simulink model "TST_ASDrf_Governor"  (R2016b)
settings: Solver=FixedStepDiscrete  StartTime=0.0  StopTime=simTime  FixedStep=sampleTime  RelTol=1e-3
values from neighbouring files (symbols this model uses):
  testCase = 1    [initTST_ASDrf_Governor_001.m]    (also in initTST_ASDrf_Governor_002.m = 2; initTST_ASDrf_Governor_003.m = 3)
libraries: simulink x10, UnitTest_Lib x6
settings Model: Creator=zhengjinyan  LastModifiedBy=zhengjinyan
settings DebuggingCC: SignalRangeChecking=error

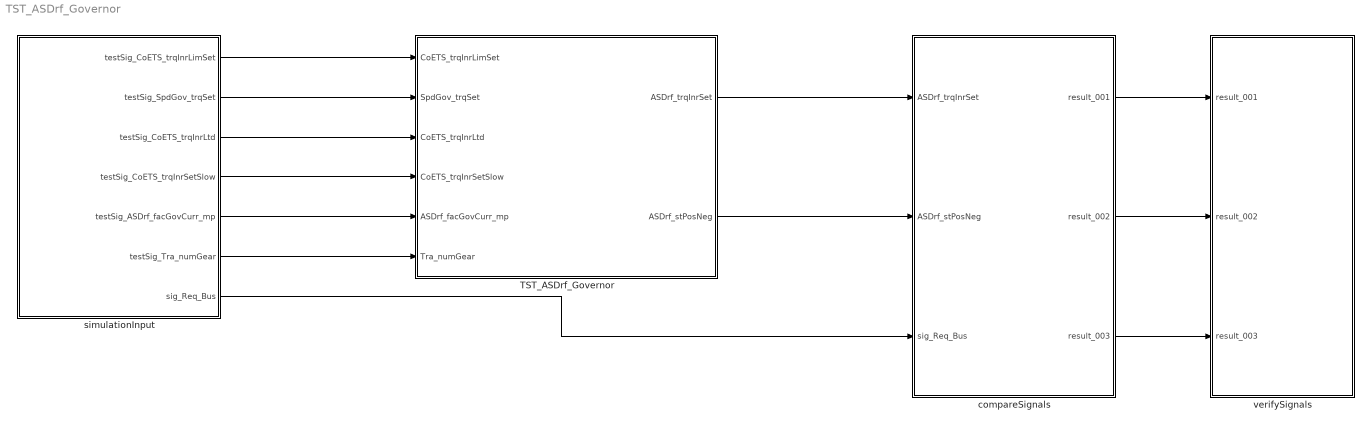
== system TST_ASDrf_Governor ==
  TST_ASDrf_Governor : Subsystem
  compareSignals : Subsystem
  simulationInput : Subsystem
  verifySignals : Subsystem
  wires:
  simulationInput/1(testSig_CoETS_trqInrLimSet) -> TST_ASDrf_Governor/1(CoETS_trqInrLimSet)
  simulationInput/2(testSig_SpdGov_trqSet) -> TST_ASDrf_Governor/2(SpdGov_trqSet)
  simulationInput/3(testSig_CoETS_trqInrLtd) -> TST_ASDrf_Governor/3(CoETS_trqInrLtd)
  simulationInput/4(testSig_CoETS_trqInrSetSlow) -> TST_ASDrf_Governor/4(CoETS_trqInrSetSlow)
  simulationInput/5(testSig_ASDrf_facGovCurr_mp) -> TST_ASDrf_Governor/5(ASDrf_facGovCurr_mp)
  simulationInput/6(testSig_Tra_numGear) -> TST_ASDrf_Governor/6(Tra_numGear)
  TST_ASDrf_Governor/1(ASDrf_trqInrSet) -> compareSignals/1(ASDrf_trqInrSet)
  TST_ASDrf_Governor/2(ASDrf_stPosNeg) -> compareSignals/2(ASDrf_stPosNeg)
  simulationInput/7(sig_Req_Bus) -> compareSignals/3(sig_Req_Bus)
  compareSignals/1(result_001) -> verifySignals/1(result_001)
  compareSignals/2(result_002) -> verifySignals/2(result_002)
  compareSignals/3(result_003) -> verifySignals/3(result_003)

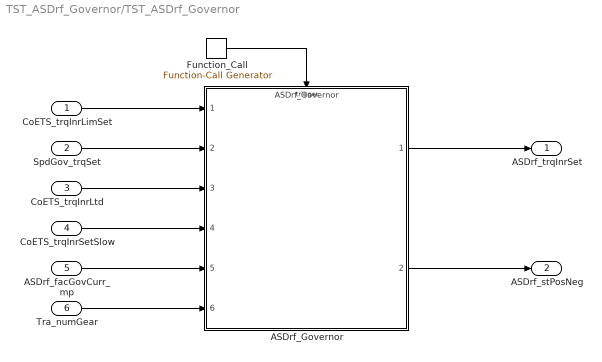
== system TST_ASDrf_Governor/TST_ASDrf_Governor ==
  CoETS_trqInrLimSet : Inport
  SpdGov_trqSet : Inport  Port=2
  CoETS_trqInrLtd : Inport  Port=3
  CoETS_trqInrSetSlow : Inport  Port=4
  ASDrf_facGovCurr_mp : Inport  Port=5
  Tra_numGear : Inport  Port=6
  ASDrf_Governor : ModelReference  ModelNameDialog=ASDrf_Governor  SimulationMode=Normal  ModelReferenceVersion=1.11  TriggerPortName=function  TriggerPortTriggerType=function-call  TriggerPortStatesWhenEnabling=held
  Function_Call : simulink/Ports & Subsystems/Function-Call Generator  sample_time=sampleTime  numberOfIterations=1
  ASDrf_trqInrSet : Outport
  ASDrf_stPosNeg : Outport  Port=2
  wires:
  Function_Call/1 -> ASDrf_Governor/Trigger
  CoETS_trqInrLimSet/1 -> ASDrf_Governor/1
  SpdGov_trqSet/1 -> ASDrf_Governor/2
  CoETS_trqInrLtd/1 -> ASDrf_Governor/3
  CoETS_trqInrSetSlow/1 -> ASDrf_Governor/4
  ASDrf_facGovCurr_mp/1 -> ASDrf_Governor/5
  Tra_numGear/1 -> ASDrf_Governor/6
  ASDrf_Governor/1 -> ASDrf_trqInrSet/1
  ASDrf_Governor/2 -> ASDrf_stPosNeg/1

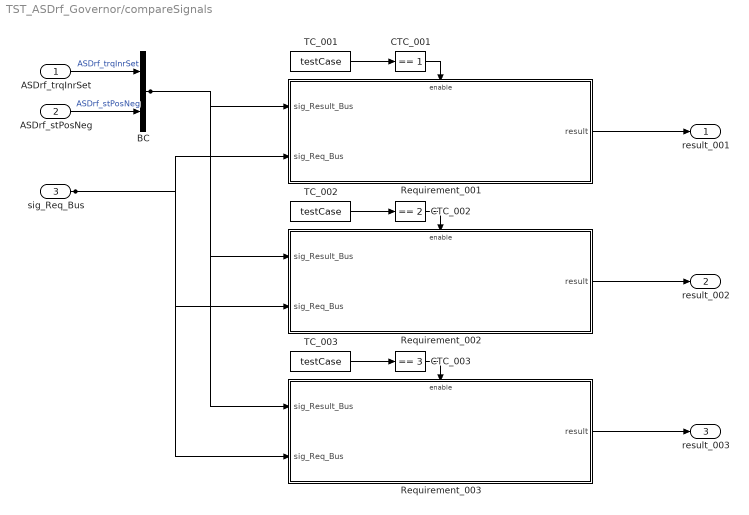
== system TST_ASDrf_Governor/compareSignals ==
  ASDrf_trqInrSet : Inport
  ASDrf_stPosNeg : Inport  Port=2
  sig_Req_Bus : Inport  Port=3
  BC : BusCreator  Inputs=2
  CTC_001 : simulink/Logic and Bit Operations/Compare To Constant  relop===  const=1  OutDataTypeStr=boolean
  CTC_002 : simulink/Logic and Bit Operations/Compare To Constant  relop===  const=2  OutDataTypeStr=boolean
  CTC_003 : simulink/Logic and Bit Operations/Compare To Constant  relop===  const=3  OutDataTypeStr=boolean
  Requirement_001 : Subsystem
  Requirement_002 : Subsystem
  Requirement_003 : Subsystem
  TC_001 : Constant  Value=testCase
  TC_002 : Constant  Value=testCase
  TC_003 : Constant  Value=testCase
  result_001 : Outport
  result_002 : Outport  Port=2
  result_003 : Outport  Port=3
  wires:
  ASDrf_trqInrSet/1 -> BC/1  "ASDrf_trqInrSet"
  ASDrf_stPosNeg/1 -> BC/2  "ASDrf_stPosNeg"
  TC_001/1 -> CTC_001/1
  CTC_001/1 -> Requirement_001/Enable
  sig_Req_Bus/1 -> Requirement_001/2(sig_Req_Bus), Requirement_002/2(sig_Req_Bus), Requirement_003/2(sig_Req_Bus)
  BC/1 -> Requirement_001/1(sig_Result_Bus), Requirement_002/1(sig_Result_Bus), Requirement_003/1(sig_Result_Bus)
  Requirement_001/1(result) -> result_001/1
  TC_002/1 -> CTC_002/1
  CTC_002/1 -> Requirement_002/Enable
  Requirement_002/1(result) -> result_002/1
  TC_003/1 -> CTC_003/1
  CTC_003/1 -> Requirement_003/Enable
  Requirement_003/1(result) -> result_003/1

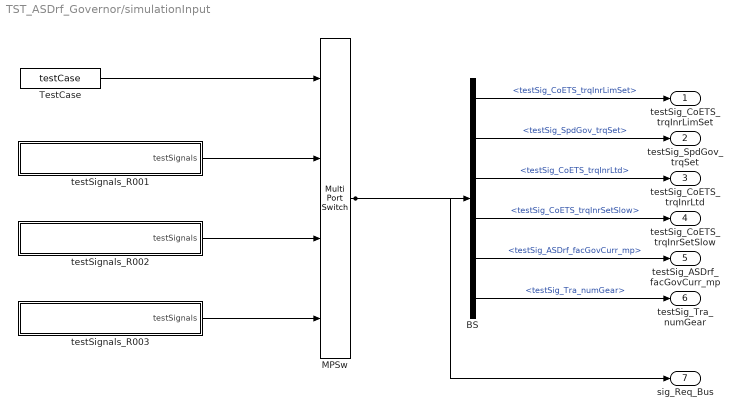
== system TST_ASDrf_Governor/simulationInput ==
  BS : BusSelector  OutputSignals=testSig_CoETS_trqInrLimSet,testSig_SpdGov_trqSet,testSig_CoETS_trqInrLtd,testSig_CoETS_trqInrSetSlow,testSig_ASDrf_facGovCurr_mp,testSig_Tra_numGear
  MPSw : MultiPortSwitch  SaturateOnIntegerOverflow=on  InputSameDT=on
  TestCase : Constant  Value=testCase
  testSignals_R001 : Subsystem
  testSignals_R002 : Subsystem
  testSignals_R003 : Subsystem
  testSig_CoETS_trqInrLimSet : Outport
  testSig_SpdGov_trqSet : Outport  Port=2
  testSig_CoETS_trqInrLtd : Outport  Port=3
  testSig_CoETS_trqInrSetSlow : Outport  Port=4
  testSig_ASDrf_facGovCurr_mp : Outport  Port=5
  testSig_Tra_numGear : Outport  Port=6
  sig_Req_Bus : Outport  Port=7
  wires:
  BS/1 -> testSig_CoETS_trqInrLimSet/1  "<testSig_CoETS_trqInrLimSet>"
  BS/2 -> testSig_SpdGov_trqSet/1  "<testSig_SpdGov_trqSet>"
  BS/3 -> testSig_CoETS_trqInrLtd/1  "<testSig_CoETS_trqInrLtd>"
  BS/4 -> testSig_CoETS_trqInrSetSlow/1  "<testSig_CoETS_trqInrSetSlow>"
  BS/5 -> testSig_ASDrf_facGovCurr_mp/1  "<testSig_ASDrf_facGovCurr_mp>"
  BS/6 -> testSig_Tra_numGear/1  "<testSig_Tra_numGear>"
  MPSw/1 -> BS/1, sig_Req_Bus/1
  TestCase/1 -> MPSw/1
  testSignals_R001/1(testSignals) -> MPSw/2
  testSignals_R002/1(testSignals) -> MPSw/3
  testSignals_R003/1(testSignals) -> MPSw/4

== system TST_ASDrf_Governor/verifySignals ==
  result_001 : Inport
  result_002 : Inport  Port=2
  result_003 : Inport  Port=3
  Assertion_001 : Assertion  Enabled=off
  Assertion_002 : Assertion  Enabled=off
  Assertion_003 : Assertion  Enabled=off
  wires:
  result_001/1 -> Assertion_001/1
  result_002/1 -> Assertion_002/1
  result_003/1 -> Assertion_003/1

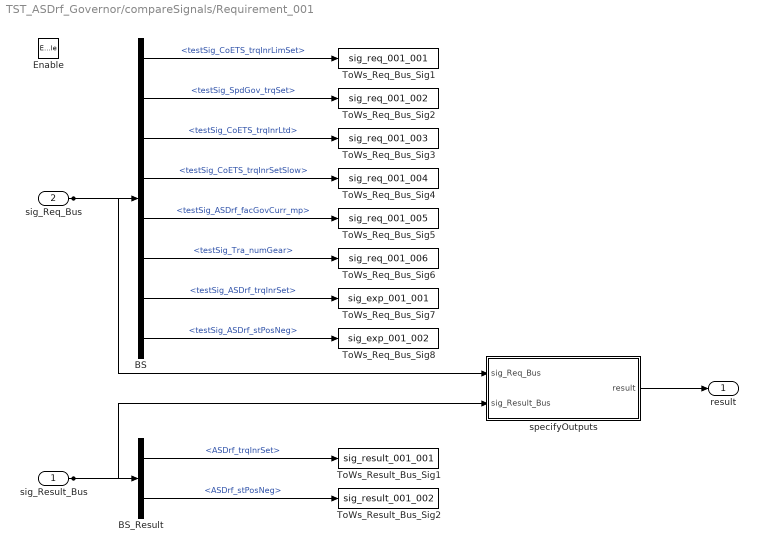
== system TST_ASDrf_Governor/compareSignals/Requirement_001 ==
  sig_Result_Bus : Inport
  sig_Req_Bus : Inport  Port=2
  Enable : EnablePort
  BS : BusSelector  OutputSignals=testSig_CoETS_trqInrLimSet,testSig_SpdGov_trqSet,testSig_CoETS_trqInrLtd,testSig_CoETS_trqInrSetSlow,testSig_ASDrf_facGovCurr_mp,testSig_Tra_numGear,testSig_ASDrf_trqInrSet,testSig_ASDrf_stPosNeg
  BS_Result : BusSelector  OutputSignals=ASDrf_trqInrSet,ASDrf_stPosNeg
  ToWs_Req_Bus_Sig1 : ToWorkspace  VariableName=sig_req_001_001  SaveFormat=Structure With Time
  ToWs_Req_Bus_Sig2 : ToWorkspace  VariableName=sig_req_001_002  SaveFormat=Structure With Time
  ToWs_Req_Bus_Sig3 : ToWorkspace  VariableName=sig_req_001_003  SaveFormat=Structure With Time
  ToWs_Req_Bus_Sig4 : ToWorkspace  VariableName=sig_req_001_004  SaveFormat=Structure With Time
  ToWs_Req_Bus_Sig5 : ToWorkspace  VariableName=sig_req_001_005  SaveFormat=Structure With Time
  ToWs_Req_Bus_Sig6 : ToWorkspace  VariableName=sig_req_001_006  SaveFormat=Structure With Time
  ToWs_Req_Bus_Sig7 : ToWorkspace  VariableName=sig_exp_001_001  SaveFormat=Structure With Time
  ToWs_Req_Bus_Sig8 : ToWorkspace  VariableName=sig_exp_001_002  SaveFormat=Structure With Time
  ToWs_Result_Bus_Sig1 : ToWorkspace  VariableName=sig_result_001_001  SaveFormat=Structure With Time
  ToWs_Result_Bus_Sig2 : ToWorkspace  VariableName=sig_result_001_002  SaveFormat=Structure With Time
  specifyOutputs : Subsystem
  result : Outport
  wires:
  sig_Req_Bus/1 -> BS/1, specifyOutputs/1(sig_Req_Bus)
  BS/1 -> ToWs_Req_Bus_Sig1/1  "<testSig_CoETS_trqInrLimSet>"
  BS/2 -> ToWs_Req_Bus_Sig2/1  "<testSig_SpdGov_trqSet>"
  BS/3 -> ToWs_Req_Bus_Sig3/1  "<testSig_CoETS_trqInrLtd>"
  BS/4 -> ToWs_Req_Bus_Sig4/1  "<testSig_CoETS_trqInrSetSlow>"
  BS/5 -> ToWs_Req_Bus_Sig5/1  "<testSig_ASDrf_facGovCurr_mp>"
  BS/6 -> ToWs_Req_Bus_Sig6/1  "<testSig_Tra_numGear>"
  BS/7 -> ToWs_Req_Bus_Sig7/1  "<testSig_ASDrf_trqInrSet>"
  BS/8 -> ToWs_Req_Bus_Sig8/1  "<testSig_ASDrf_stPosNeg>"
  sig_Result_Bus/1 -> BS_Result/1, specifyOutputs/2(sig_Result_Bus)
  BS_Result/1 -> ToWs_Result_Bus_Sig1/1  "<ASDrf_trqInrSet>"
  BS_Result/2 -> ToWs_Result_Bus_Sig2/1  "<ASDrf_stPosNeg>"
  specifyOutputs/1(result) -> result/1

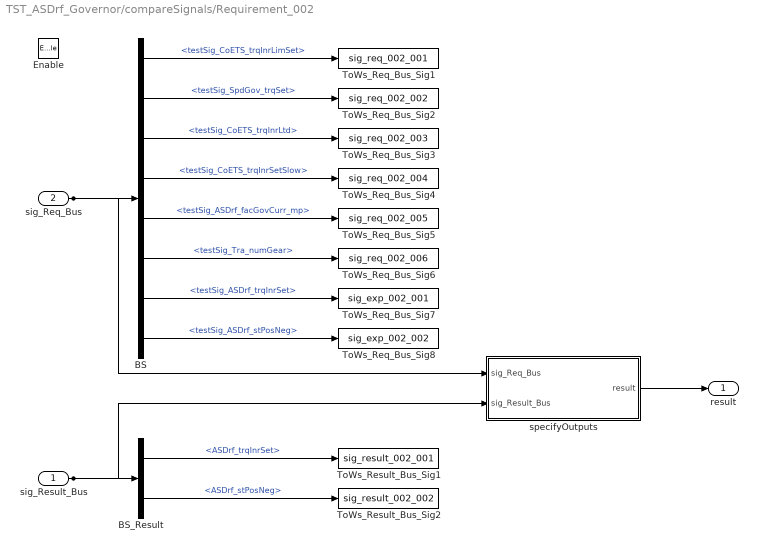
== system TST_ASDrf_Governor/compareSignals/Requirement_002 ==
  sig_Result_Bus : Inport
  sig_Req_Bus : Inport  Port=2
  Enable : EnablePort
  BS : BusSelector  OutputSignals=testSig_CoETS_trqInrLimSet,testSig_SpdGov_trqSet,testSig_CoETS_trqInrLtd,testSig_CoETS_trqInrSetSlow,testSig_ASDrf_facGovCurr_mp,testSig_Tra_numGear,testSig_ASDrf_trqInrSet,testSig_ASDrf_stPosNeg
  BS_Result : BusSelector  OutputSignals=ASDrf_trqInrSet,ASDrf_stPosNeg
  ToWs_Req_Bus_Sig1 : ToWorkspace  VariableName=sig_req_002_001  SaveFormat=Structure With Time
  ToWs_Req_Bus_Sig2 : ToWorkspace  VariableName=sig_req_002_002  SaveFormat=Structure With Time
  ToWs_Req_Bus_Sig3 : ToWorkspace  VariableName=sig_req_002_003  SaveFormat=Structure With Time
  ToWs_Req_Bus_Sig4 : ToWorkspace  VariableName=sig_req_002_004  SaveFormat=Structure With Time
  ToWs_Req_Bus_Sig5 : ToWorkspace  VariableName=sig_req_002_005  SaveFormat=Structure With Time
  ToWs_Req_Bus_Sig6 : ToWorkspace  VariableName=sig_req_002_006  SaveFormat=Structure With Time
  ToWs_Req_Bus_Sig7 : ToWorkspace  VariableName=sig_exp_002_001  SaveFormat=Structure With Time
  ToWs_Req_Bus_Sig8 : ToWorkspace  VariableName=sig_exp_002_002  SaveFormat=Structure With Time
  ToWs_Result_Bus_Sig1 : ToWorkspace  VariableName=sig_result_002_001  SaveFormat=Structure With Time
  ToWs_Result_Bus_Sig2 : ToWorkspace  VariableName=sig_result_002_002  SaveFormat=Structure With Time
  specifyOutputs : Subsystem
  result : Outport
  wires:
  sig_Req_Bus/1 -> BS/1, specifyOutputs/1(sig_Req_Bus)
  BS/1 -> ToWs_Req_Bus_Sig1/1  "<testSig_CoETS_trqInrLimSet>"
  BS/2 -> ToWs_Req_Bus_Sig2/1  "<testSig_SpdGov_trqSet>"
  BS/3 -> ToWs_Req_Bus_Sig3/1  "<testSig_CoETS_trqInrLtd>"
  BS/4 -> ToWs_Req_Bus_Sig4/1  "<testSig_CoETS_trqInrSetSlow>"
  BS/5 -> ToWs_Req_Bus_Sig5/1  "<testSig_ASDrf_facGovCurr_mp>"
  BS/6 -> ToWs_Req_Bus_Sig6/1  "<testSig_Tra_numGear>"
  BS/7 -> ToWs_Req_Bus_Sig7/1  "<testSig_ASDrf_trqInrSet>"
  BS/8 -> ToWs_Req_Bus_Sig8/1  "<testSig_ASDrf_stPosNeg>"
  sig_Result_Bus/1 -> BS_Result/1, specifyOutputs/2(sig_Result_Bus)
  BS_Result/1 -> ToWs_Result_Bus_Sig1/1  "<ASDrf_trqInrSet>"
  BS_Result/2 -> ToWs_Result_Bus_Sig2/1  "<ASDrf_stPosNeg>"
  specifyOutputs/1(result) -> result/1

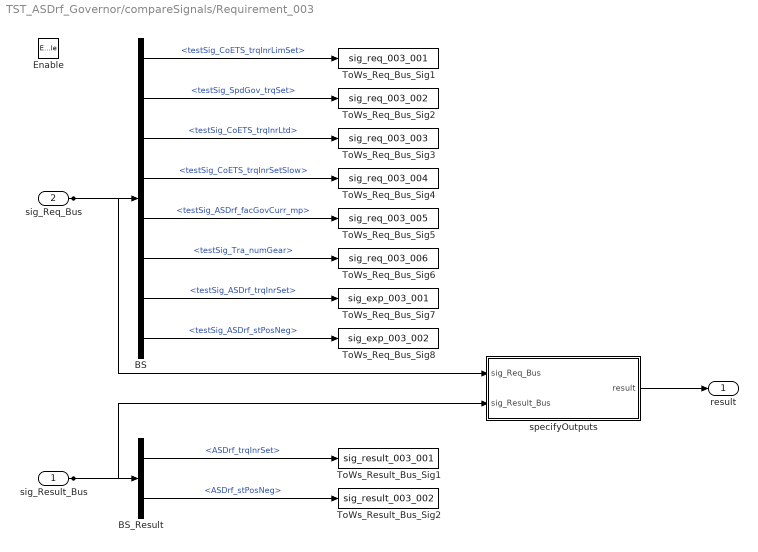
== system TST_ASDrf_Governor/compareSignals/Requirement_003 ==
  sig_Result_Bus : Inport
  sig_Req_Bus : Inport  Port=2
  Enable : EnablePort
  BS : BusSelector  OutputSignals=testSig_CoETS_trqInrLimSet,testSig_SpdGov_trqSet,testSig_CoETS_trqInrLtd,testSig_CoETS_trqInrSetSlow,testSig_ASDrf_facGovCurr_mp,testSig_Tra_numGear,testSig_ASDrf_trqInrSet,testSig_ASDrf_stPosNeg
  BS_Result : BusSelector  OutputSignals=ASDrf_trqInrSet,ASDrf_stPosNeg
  ToWs_Req_Bus_Sig1 : ToWorkspace  VariableName=sig_req_003_001  SaveFormat=Structure With Time
  ToWs_Req_Bus_Sig2 : ToWorkspace  VariableName=sig_req_003_002  SaveFormat=Structure With Time
  ToWs_Req_Bus_Sig3 : ToWorkspace  VariableName=sig_req_003_003  SaveFormat=Structure With Time
  ToWs_Req_Bus_Sig4 : ToWorkspace  VariableName=sig_req_003_004  SaveFormat=Structure With Time
  ToWs_Req_Bus_Sig5 : ToWorkspace  VariableName=sig_req_003_005  SaveFormat=Structure With Time
  ToWs_Req_Bus_Sig6 : ToWorkspace  VariableName=sig_req_003_006  SaveFormat=Structure With Time
  ToWs_Req_Bus_Sig7 : ToWorkspace  VariableName=sig_exp_003_001  SaveFormat=Structure With Time
  ToWs_Req_Bus_Sig8 : ToWorkspace  VariableName=sig_exp_003_002  SaveFormat=Structure With Time
  ToWs_Result_Bus_Sig1 : ToWorkspace  VariableName=sig_result_003_001  SaveFormat=Structure With Time
  ToWs_Result_Bus_Sig2 : ToWorkspace  VariableName=sig_result_003_002  SaveFormat=Structure With Time
  specifyOutputs : Subsystem
  result : Outport
  wires:
  sig_Req_Bus/1 -> BS/1, specifyOutputs/1(sig_Req_Bus)
  BS/1 -> ToWs_Req_Bus_Sig1/1  "<testSig_CoETS_trqInrLimSet>"
  BS/2 -> ToWs_Req_Bus_Sig2/1  "<testSig_SpdGov_trqSet>"
  BS/3 -> ToWs_Req_Bus_Sig3/1  "<testSig_CoETS_trqInrLtd>"
  BS/4 -> ToWs_Req_Bus_Sig4/1  "<testSig_CoETS_trqInrSetSlow>"
  BS/5 -> ToWs_Req_Bus_Sig5/1  "<testSig_ASDrf_facGovCurr_mp>"
  BS/6 -> ToWs_Req_Bus_Sig6/1  "<testSig_Tra_numGear>"
  BS/7 -> ToWs_Req_Bus_Sig7/1  "<testSig_ASDrf_trqInrSet>"
  BS/8 -> ToWs_Req_Bus_Sig8/1  "<testSig_ASDrf_stPosNeg>"
  sig_Result_Bus/1 -> BS_Result/1, specifyOutputs/2(sig_Result_Bus)
  BS_Result/1 -> ToWs_Result_Bus_Sig1/1  "<ASDrf_trqInrSet>"
  BS_Result/2 -> ToWs_Result_Bus_Sig2/1  "<ASDrf_stPosNeg>"
  specifyOutputs/1(result) -> result/1

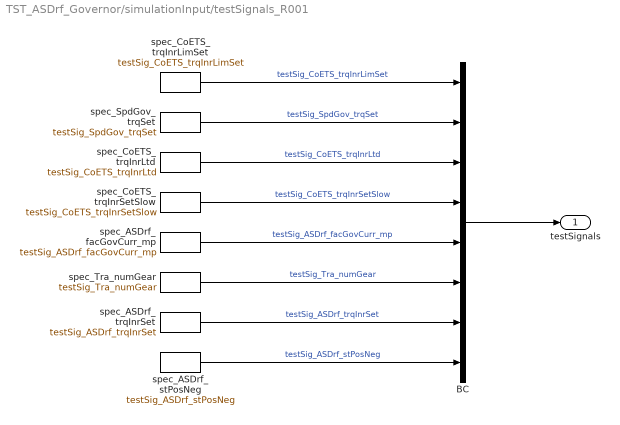
== system TST_ASDrf_Governor/simulationInput/testSignals_R001 ==
  BC : BusCreator  Inputs=8
  spec_ASDrf_facGovCurr_mp : FromWorkspace  VariableName=testSig_ASDrf_facGovCurr_mp  Interpolate=off  OutputAfterFinalValue=Holding final value
  spec_ASDrf_stPosNeg : FromWorkspace  VariableName=testSig_ASDrf_stPosNeg  Interpolate=off  OutputAfterFinalValue=Holding final value
  spec_ASDrf_trqInrSet : FromWorkspace  VariableName=testSig_ASDrf_trqInrSet  Interpolate=off  OutputAfterFinalValue=Holding final value
  spec_CoETS_trqInrLimSet : FromWorkspace  VariableName=testSig_CoETS_trqInrLimSet  Interpolate=off  OutputAfterFinalValue=Holding final value
  spec_CoETS_trqInrLtd : FromWorkspace  VariableName=testSig_CoETS_trqInrLtd  Interpolate=off  OutputAfterFinalValue=Holding final value
  spec_CoETS_trqInrSetSlow : FromWorkspace  VariableName=testSig_CoETS_trqInrSetSlow  Interpolate=off  OutputAfterFinalValue=Holding final value
  spec_SpdGov_trqSet : FromWorkspace  VariableName=testSig_SpdGov_trqSet  Interpolate=off  OutputAfterFinalValue=Holding final value
  spec_Tra_numGear : FromWorkspace  VariableName=testSig_Tra_numGear  Interpolate=off  OutputAfterFinalValue=Holding final value
  testSignals : Outport
  wires:
  BC/1 -> testSignals/1
  spec_CoETS_trqInrLimSet/1 -> BC/1  "testSig_CoETS_trqInrLimSet"
  spec_SpdGov_trqSet/1 -> BC/2  "testSig_SpdGov_trqSet"
  spec_CoETS_trqInrLtd/1 -> BC/3  "testSig_CoETS_trqInrLtd"
  spec_CoETS_trqInrSetSlow/1 -> BC/4  "testSig_CoETS_trqInrSetSlow"
  spec_ASDrf_facGovCurr_mp/1 -> BC/5  "testSig_ASDrf_facGovCurr_mp"
  spec_Tra_numGear/1 -> BC/6  "testSig_Tra_numGear"
  spec_ASDrf_trqInrSet/1 -> BC/7  "testSig_ASDrf_trqInrSet"
  spec_ASDrf_stPosNeg/1 -> BC/8  "testSig_ASDrf_stPosNeg"

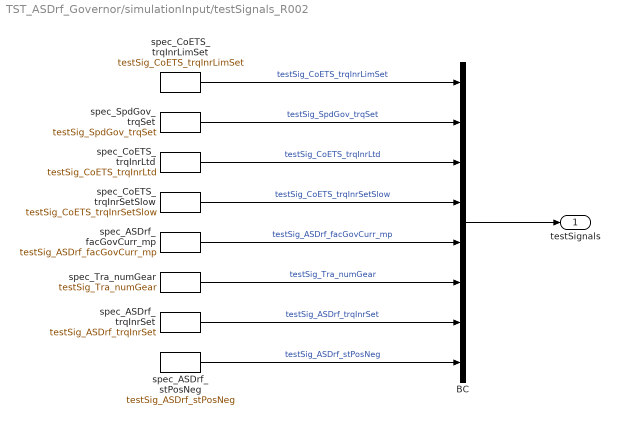
== system TST_ASDrf_Governor/simulationInput/testSignals_R002 ==
  BC : BusCreator  Inputs=8
  spec_ASDrf_facGovCurr_mp : FromWorkspace  VariableName=testSig_ASDrf_facGovCurr_mp  Interpolate=off  OutputAfterFinalValue=Holding final value
  spec_ASDrf_stPosNeg : FromWorkspace  VariableName=testSig_ASDrf_stPosNeg  Interpolate=off  OutputAfterFinalValue=Holding final value
  spec_ASDrf_trqInrSet : FromWorkspace  VariableName=testSig_ASDrf_trqInrSet  Interpolate=off  OutputAfterFinalValue=Holding final value
  spec_CoETS_trqInrLimSet : FromWorkspace  VariableName=testSig_CoETS_trqInrLimSet  Interpolate=off  OutputAfterFinalValue=Holding final value
  spec_CoETS_trqInrLtd : FromWorkspace  VariableName=testSig_CoETS_trqInrLtd  Interpolate=off  OutputAfterFinalValue=Holding final value
  spec_CoETS_trqInrSetSlow : FromWorkspace  VariableName=testSig_CoETS_trqInrSetSlow  Interpolate=off  OutputAfterFinalValue=Holding final value
  spec_SpdGov_trqSet : FromWorkspace  VariableName=testSig_SpdGov_trqSet  Interpolate=off  OutputAfterFinalValue=Holding final value
  spec_Tra_numGear : FromWorkspace  VariableName=testSig_Tra_numGear  Interpolate=off  OutputAfterFinalValue=Holding final value
  testSignals : Outport
  wires:
  BC/1 -> testSignals/1
  spec_CoETS_trqInrLimSet/1 -> BC/1  "testSig_CoETS_trqInrLimSet"
  spec_SpdGov_trqSet/1 -> BC/2  "testSig_SpdGov_trqSet"
  spec_CoETS_trqInrLtd/1 -> BC/3  "testSig_CoETS_trqInrLtd"
  spec_CoETS_trqInrSetSlow/1 -> BC/4  "testSig_CoETS_trqInrSetSlow"
  spec_ASDrf_facGovCurr_mp/1 -> BC/5  "testSig_ASDrf_facGovCurr_mp"
  spec_Tra_numGear/1 -> BC/6  "testSig_Tra_numGear"
  spec_ASDrf_trqInrSet/1 -> BC/7  "testSig_ASDrf_trqInrSet"
  spec_ASDrf_stPosNeg/1 -> BC/8  "testSig_ASDrf_stPosNeg"

== system TST_ASDrf_Governor/simulationInput/testSignals_R003 ==
  BC : BusCreator  Inputs=8
  spec_ASDrf_facGovCurr_mp : FromWorkspace  VariableName=testSig_ASDrf_facGovCurr_mp  Interpolate=off  OutputAfterFinalValue=Holding final value
  spec_ASDrf_stPosNeg : FromWorkspace  VariableName=testSig_ASDrf_stPosNeg  Interpolate=off  OutputAfterFinalValue=Holding final value
  spec_ASDrf_trqInrSet : FromWorkspace  VariableName=testSig_ASDrf_trqInrSet  Interpolate=off  OutputAfterFinalValue=Holding final value
  spec_CoETS_trqInrLimSet : FromWorkspace  VariableName=testSig_CoETS_trqInrLimSet  Interpolate=off  OutputAfterFinalValue=Holding final value
  spec_CoETS_trqInrLtd : FromWorkspace  VariableName=testSig_CoETS_trqInrLtd  Interpolate=off  OutputAfterFinalValue=Holding final value
  spec_CoETS_trqInrSetSlow : FromWorkspace  VariableName=testSig_CoETS_trqInrSetSlow  Interpolate=off  OutputAfterFinalValue=Holding final value
  spec_SpdGov_trqSet : FromWorkspace  VariableName=testSig_SpdGov_trqSet  Interpolate=off  OutputAfterFinalValue=Holding final value
  spec_Tra_numGear : FromWorkspace  VariableName=testSig_Tra_numGear  Interpolate=off  OutputAfterFinalValue=Holding final value
  testSignals : Outport
  wires:
  BC/1 -> testSignals/1
  spec_CoETS_trqInrLimSet/1 -> BC/1  "testSig_CoETS_trqInrLimSet"
  spec_SpdGov_trqSet/1 -> BC/2  "testSig_SpdGov_trqSet"
  spec_CoETS_trqInrLtd/1 -> BC/3  "testSig_CoETS_trqInrLtd"
  spec_CoETS_trqInrSetSlow/1 -> BC/4  "testSig_CoETS_trqInrSetSlow"
  spec_ASDrf_facGovCurr_mp/1 -> BC/5  "testSig_ASDrf_facGovCurr_mp"
  spec_Tra_numGear/1 -> BC/6  "testSig_Tra_numGear"
  spec_ASDrf_trqInrSet/1 -> BC/7  "testSig_ASDrf_trqInrSet"
  spec_ASDrf_stPosNeg/1 -> BC/8  "testSig_ASDrf_stPosNeg"

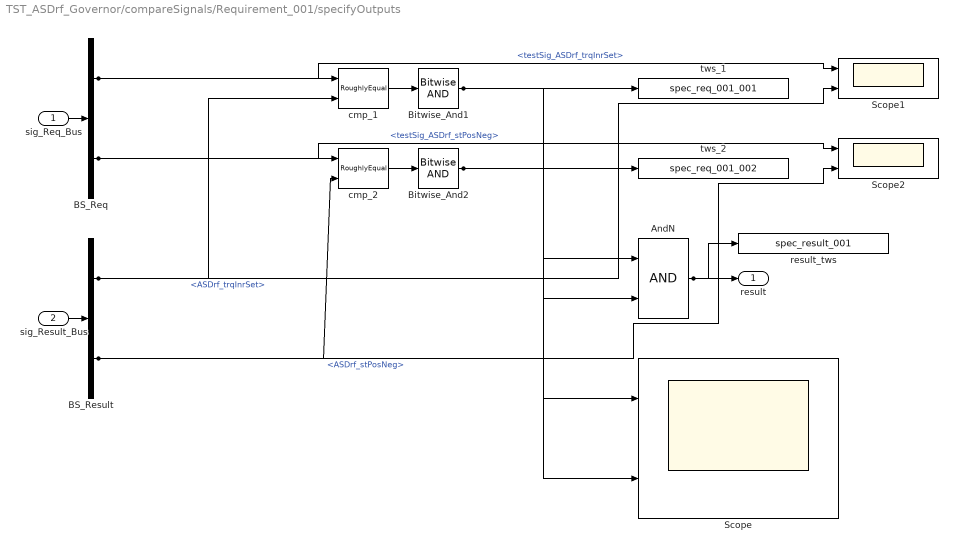
== system TST_ASDrf_Governor/compareSignals/Requirement_001/specifyOutputs ==
  sig_Req_Bus : Inport
  sig_Result_Bus : Inport  Port=2
  AndN : Logic
  BS_Req : BusSelector  OutputSignals=testSig_ASDrf_trqInrSet,testSig_ASDrf_stPosNeg
  BS_Result : BusSelector  OutputSignals=ASDrf_trqInrSet,ASDrf_stPosNeg
  Bitwise_And1 : simulink/Logic and Bit Operations/Bitwise Operator  logicop=AND  UseBitMask=off  BitMask=bin2dec('11011001')  BitMaskRealWorld=Stored Integer
  Bitwise_And2 : simulink/Logic and Bit Operations/Bitwise Operator  logicop=AND  UseBitMask=off  BitMask=bin2dec('11011001')  BitMaskRealWorld=Stored Integer
  Scope : Scope  NumInputPorts=2
  Scope1 : Scope  NumInputPorts=2
  Scope2 : Scope  NumInputPorts=2
  cmp_1 : UnitTest_Lib/RoughlyEqual  slope=0.1
  cmp_2 : UnitTest_Lib/RoughlyEqual  slope=0.1
  result_tws : ToWorkspace  VariableName=spec_result_001
  tws_1 : ToWorkspace  VariableName=spec_req_001_001
  tws_2 : ToWorkspace  VariableName=spec_req_001_002
  result : Outport
  wires:
  sig_Req_Bus/1 -> BS_Req/1
  sig_Result_Bus/1 -> BS_Result/1
  AndN/1 -> result/1, result_tws/1
  BS_Req/1 -> cmp_1/1, Scope1/1  "<testSig_ASDrf_trqInrSet>"
  BS_Result/1 -> cmp_1/2, Scope1/2  "<ASDrf_trqInrSet>"
  cmp_1/1 -> Bitwise_And1/1
  Bitwise_And1/1 -> tws_1/1, AndN/1, Scope/1
  BS_Req/2 -> cmp_2/1, Scope2/1  "<testSig_ASDrf_stPosNeg>"
  BS_Result/2 -> cmp_2/2, Scope2/2  "<ASDrf_stPosNeg>"
  cmp_2/1 -> Bitwise_And2/1
  Bitwise_And2/1 -> tws_2/1, AndN/2, Scope/2

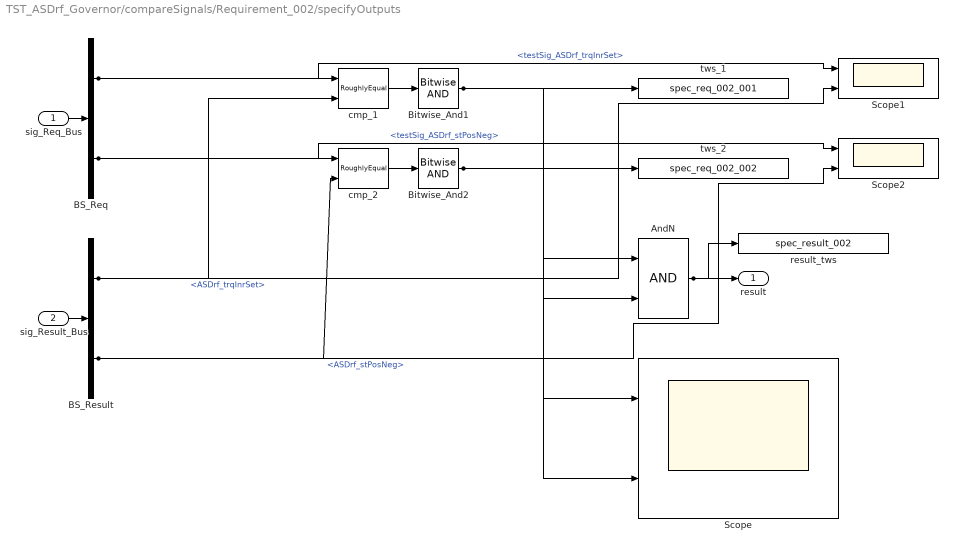
== system TST_ASDrf_Governor/compareSignals/Requirement_002/specifyOutputs ==
  sig_Req_Bus : Inport
  sig_Result_Bus : Inport  Port=2
  AndN : Logic
  BS_Req : BusSelector  OutputSignals=testSig_ASDrf_trqInrSet,testSig_ASDrf_stPosNeg
  BS_Result : BusSelector  OutputSignals=ASDrf_trqInrSet,ASDrf_stPosNeg
  Bitwise_And1 : simulink/Logic and Bit Operations/Bitwise Operator  logicop=AND  UseBitMask=off  BitMask=bin2dec('11011001')  BitMaskRealWorld=Stored Integer
  Bitwise_And2 : simulink/Logic and Bit Operations/Bitwise Operator  logicop=AND  UseBitMask=off  BitMask=bin2dec('11011001')  BitMaskRealWorld=Stored Integer
  Scope : Scope  NumInputPorts=2
  Scope1 : Scope  NumInputPorts=2
  Scope2 : Scope  NumInputPorts=2
  cmp_1 : UnitTest_Lib/RoughlyEqual  slope=0.1
  cmp_2 : UnitTest_Lib/RoughlyEqual  slope=0.1
  result_tws : ToWorkspace  VariableName=spec_result_002
  tws_1 : ToWorkspace  VariableName=spec_req_002_001
  tws_2 : ToWorkspace  VariableName=spec_req_002_002
  result : Outport
  wires:
  sig_Req_Bus/1 -> BS_Req/1
  sig_Result_Bus/1 -> BS_Result/1
  AndN/1 -> result/1, result_tws/1
  BS_Req/1 -> cmp_1/1, Scope1/1  "<testSig_ASDrf_trqInrSet>"
  BS_Result/1 -> cmp_1/2, Scope1/2  "<ASDrf_trqInrSet>"
  cmp_1/1 -> Bitwise_And1/1
  Bitwise_And1/1 -> tws_1/1, AndN/1, Scope/1
  BS_Req/2 -> cmp_2/1, Scope2/1  "<testSig_ASDrf_stPosNeg>"
  BS_Result/2 -> cmp_2/2, Scope2/2  "<ASDrf_stPosNeg>"
  cmp_2/1 -> Bitwise_And2/1
  Bitwise_And2/1 -> tws_2/1, AndN/2, Scope/2

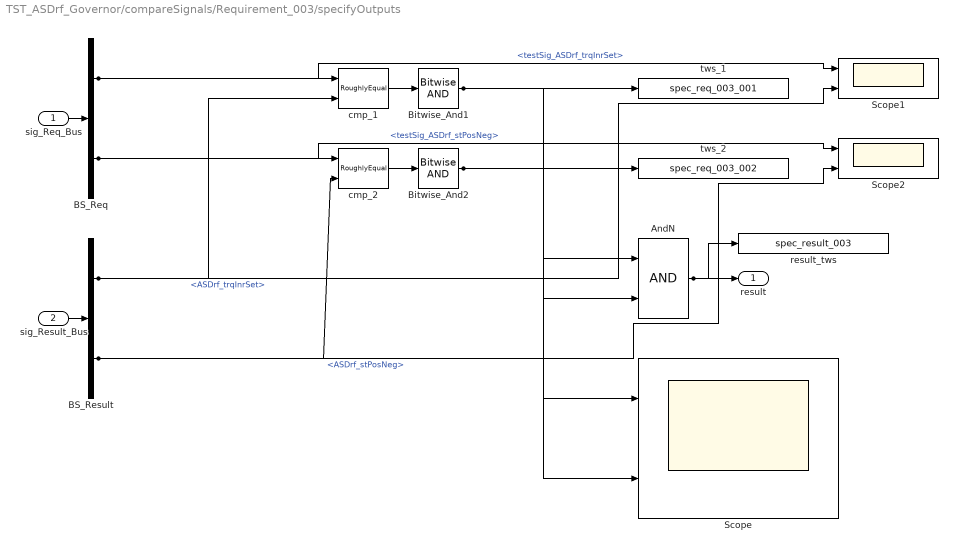
== system TST_ASDrf_Governor/compareSignals/Requirement_003/specifyOutputs ==
  sig_Req_Bus : Inport
  sig_Result_Bus : Inport  Port=2
  AndN : Logic
  BS_Req : BusSelector  OutputSignals=testSig_ASDrf_trqInrSet,testSig_ASDrf_stPosNeg
  BS_Result : BusSelector  OutputSignals=ASDrf_trqInrSet,ASDrf_stPosNeg
  Bitwise_And1 : simulink/Logic and Bit Operations/Bitwise Operator  logicop=AND  UseBitMask=off  BitMask=bin2dec('11011001')  BitMaskRealWorld=Stored Integer
  Bitwise_And2 : simulink/Logic and Bit Operations/Bitwise Operator  logicop=AND  UseBitMask=off  BitMask=bin2dec('11011001')  BitMaskRealWorld=Stored Integer
  Scope : Scope  NumInputPorts=2
  Scope1 : Scope  NumInputPorts=2
  Scope2 : Scope  NumInputPorts=2
  cmp_1 : UnitTest_Lib/RoughlyEqual  slope=0.1
  cmp_2 : UnitTest_Lib/RoughlyEqual  slope=0.1
  result_tws : ToWorkspace  VariableName=spec_result_003
  tws_1 : ToWorkspace  VariableName=spec_req_003_001
  tws_2 : ToWorkspace  VariableName=spec_req_003_002
  result : Outport
  wires:
  sig_Req_Bus/1 -> BS_Req/1
  sig_Result_Bus/1 -> BS_Result/1
  AndN/1 -> result/1, result_tws/1
  BS_Req/1 -> cmp_1/1, Scope1/1  "<testSig_ASDrf_trqInrSet>"
  BS_Result/1 -> cmp_1/2, Scope1/2  "<ASDrf_trqInrSet>"
  cmp_1/1 -> Bitwise_And1/1
  Bitwise_And1/1 -> tws_1/1, AndN/1, Scope/1
  BS_Req/2 -> cmp_2/1, Scope2/1  "<testSig_ASDrf_stPosNeg>"
  BS_Result/2 -> cmp_2/2, Scope2/2  "<ASDrf_stPosNeg>"
  cmp_2/1 -> Bitwise_And2/1
  Bitwise_And2/1 -> tws_2/1, AndN/2, Scope/2
